simulink model "PilotModelUnitTest"  (R2018b)
settings: Solver=VariableStepAuto  StartTime=0.0  StopTime=100  RelTol=1e-3
values from neighbouring files (symbols this model uses):
  enableHorzMan = 1    [unitTest_PilotModel.m]
  enableVertMan = 0    [unitTest_PilotModel.m]
undefined symbols (not defined in the file or in its folder): ac2dyn_alt0_ft, ac2dyn_con, ac2dyn_lat0_rad, ac2dyn_lon0_rad, daaLogic_turnRate_dps, daaLogic_vertRate_fpm, ddh_ftps2, dh_ftps, dv_ftps2, e_ft, Edot_ftps, h_ft, hdot_ftps, latLonAltState, n_ft, Ndot_ftps, p_radps, phi_rad, phidot_radps, psi_rad, psidot_radps, q_radps, r_radps, theta_rad, thetadot_radps, uasPilot_altitudeK, uasPilot_altitudeOffset, uasPilot_altitudeTheta, uasPilot_coordDelayK, uasPilot_coordDelayMin, uasPilot_coordDelayTheta, uasPilot_desiredTurnRate_dps, uasPilot_desiredVertRate_ftpm, uasPilot_deterministicMode, uasPilot_dt_s, uasPilot_executionDelayMin, uasPilot_executionDelayMu, uasPilot_initialDelayMin, uasPilot_initialDelayMu, uasPilot_maxRelativeHdg, uasPilot_meanUpdateTimes, uasPilot_mentalFilter_climbThresh_fps, uasPilot_mentalFilter_numSamp, uasPilot_mentalFilter_turnThresh_rad, uasPilot_minUpdateTimes, uasPilot_operatorEnabled, uasPilot_probDescend, uasPilot_probFollowMinDev, uasPilot_probLeftTurn, uasPilot_probTurn, uasPilot_reducedClimbAlt_ft, uasPilot_reducedTurnAngle_deg, uasPilot_seedChoose, uasPilot_seedCoordDelay, uasPilot_seedExecutionDelay, uasPilot_seedInitialDelay, uasPilot_seedTurn, uasPilot_seedUpdate, uasPilot_seedVertical, uasPilot_triggerLevel ... (+8)
libraries: simulink x17, NullAircraftEstimateBus x1, uas_pilot_model_r6 x1
(part 2 of 2)

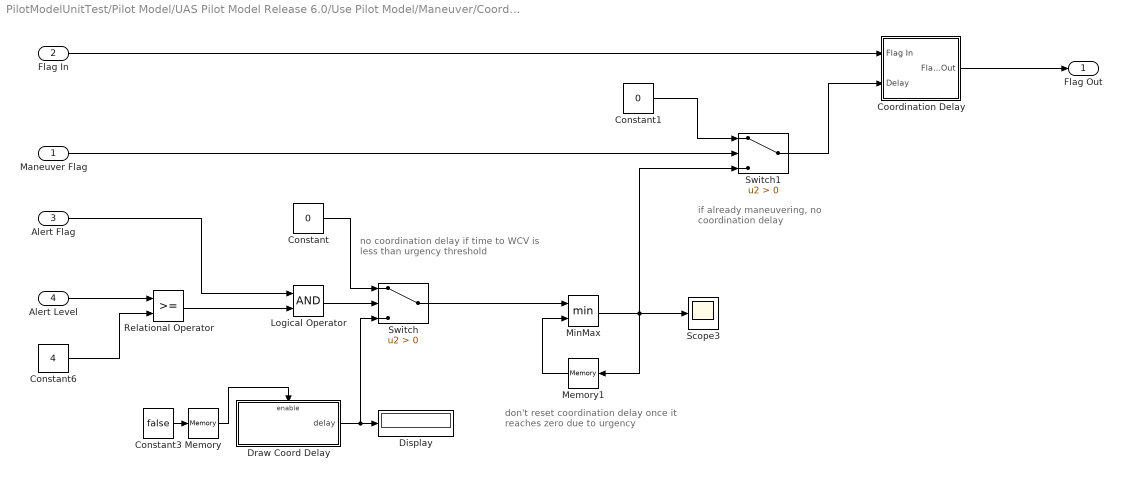
== system PilotModelUnitTest/Pilot Model/UAS Pilot Model Release 6.0/Use Pilot Model/Maneuver/Coordination Delay ==
  note: don't reset coordination delay once
      | it reaches zero due to urgency
  note: no coordination delay if time to WCV
      | is less than urgency threshold
  note: if already maneuvering, no
      | coordination delay
  Maneuver Flag : Inport
  Flag In : Inport  Port=2
  Alert Flag : Inport  Port=3
  Alert Level : Inport  Port=4
  Constant : Constant  Value=0
  Constant1 : Constant  Value=0
  Constant3 : Constant  Value=false
  Constant6 : Constant  Value=4
  Coordination Delay : Subsystem
  Display : Display
  Draw Coord Delay : Subsystem  TreatAsAtomicUnit=on  mask{k=coord_delay_k, theta=coord_delay_theta, offset=coord_delay_min, seed=rng_seed_coord}
      mask prompts: k "Gamma Distribution Shape Parameter, k"; theta "Gamma Distribution Scale Parameter, theta"
  Logical Operator : Logic  AllPortsSameDT=off  OutDataTypeStr=boolean
  Memory : Memory  InitialCondition=true  InheritSampleTime=on
  Memory1 : Memory  InitialCondition=1000  InheritSampleTime=on
  MinMax : MinMax  Inputs=2
  Relational Operator : RelationalOperator  OutDataTypeStr=boolean  RndMeth=Nearest
  Scope3 : Scope
  Switch : Switch  Criteria=u2 > Threshold
  Switch1 : Switch  Criteria=u2 > Threshold
  Flag Out : Outport
  wires:
  Constant3/1 -> Memory/1
  Memory/1 -> Draw Coord Delay/Enable
  Maneuver Flag/1 -> Switch1/2
  Constant1/1 -> Switch1/1
  Switch1/1 -> Coordination Delay/2(Delay)
  Constant/1 -> Switch/1
  Alert Level/1 -> Relational Operator/1
  Coordination Delay/1(Flag Out) -> Flag Out/1
  Relational Operator/1 -> Logical Operator/2
  Constant6/1 -> Relational Operator/2
  Logical Operator/1 -> Switch/2
  Draw Coord Delay/1(delay) -> Switch/3, Display/1
  MinMax/1 -> Memory1/1, Scope3/1, Switch1/3
  Memory1/1 -> MinMax/2
  Switch/1 -> MinMax/1
  Flag In/1 -> Coordination Delay/1(Flag In)
  Alert Flag/1 -> Logical Operator/1

== system PilotModelUnitTest/Pilot Model/UAS Pilot Model Release 6.0/Use Pilot Model/Maneuver/Initial Delay ==
  note: If already maneuvering, no delay
      | for subsequent maneuvers
  Maneuver Flag : Inport
  Alert Flag : Inport  Port=2
  Constant1 : Constant  Value=0
  Constant3 : Constant  Value=false
  Display : Display
  Draw Initial Delay : Subsystem  TreatAsAtomicUnit=on  mask{mu=mean_initial_delay, offset=min_initial_delay, seed=rng_seed_initial}
      mask prompts: mu "Exponential Distribution Mean Parameter, k"
  Memory : Memory  InitialCondition=true  InheritSampleTime=on
  Scope : Scope  NumInputPorts=2
  Switch1 : Switch  Criteria=u2 > Threshold
  Wait for Intruder to Give Way : Subsystem
  Flag Out : Outport
  wires:
  Constant3/1 -> Memory/1
  Memory/1 -> Draw Initial Delay/Enable
  Constant1/1 -> Switch1/1
  Draw Initial Delay/1(delay) -> Display/1, Switch1/3
  Switch1/1 -> Wait for Intruder to Give Way/2(Delay)
  Maneuver Flag/1 -> Switch1/2
  Wait for Intruder to Give Way/1(Flag Out) -> Scope/2, Flag Out/1
  Alert Flag/1 -> Scope/1, Wait for Intruder to Give Way/1(Flag In)

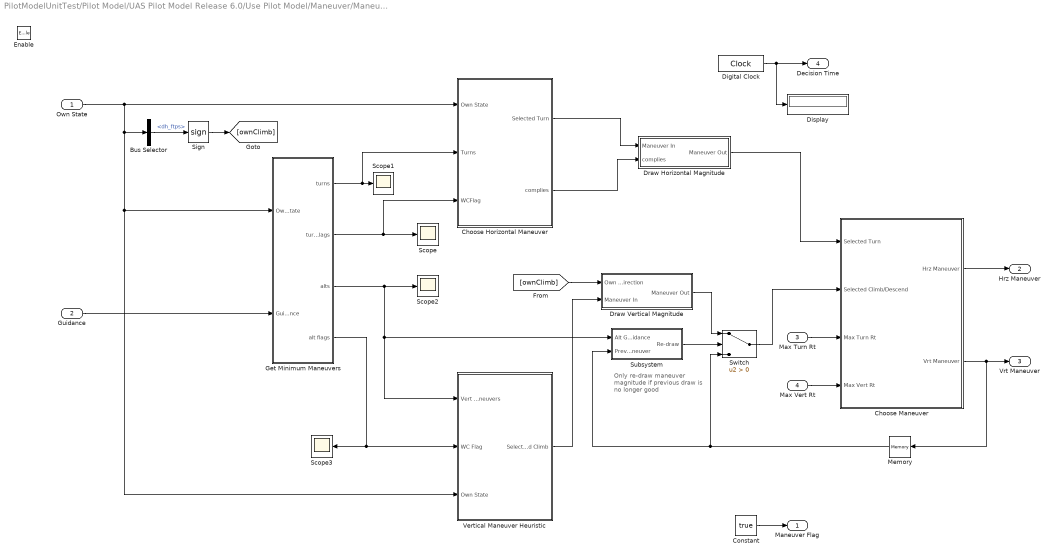
== system PilotModelUnitTest/Pilot Model/UAS Pilot Model Release 6.0/Use Pilot Model/Maneuver/Maneuver Selection ==
  note: Only re-draw maneuver
      | magnitude if previous
      | draw is no longer good
  Own State : Inport
  Guidance : Inport  Port=2
  Max Turn Rt : Inport  Port=3
  Max Vert Rt : Inport  Port=4
  Enable : EnablePort
  Bus Selector : BusSelector  OutputSignals=dh_ftps
  Choose Horizontal Maneuver : Subsystem
  Choose Maneuver : Subsystem
  Constant : Constant  Value=true
  Digital Clock : DigitalClock
  Display : Display
  Draw Horizontal Magnitude : Subsystem
  Draw Vertical Magnitude : Subsystem
  Get Minimum Maneuvers : Subsystem
  Memory : Memory  InheritSampleTime=on
  Scope{,1..3} (4 alike) : Scope
  Sign : Signum
  Subsystem : Subsystem
  Switch : Switch  Criteria=u2 > Threshold
  Vertical Maneuver Heuristic : Subsystem
  Maneuver Flag : Outport  InitialOutput=0
  Hrz Maneuver : Outport  Port=2  OutDataTypeStr=Bus: AvoidanceManeuver  InitialOutput=0
  Vrt Maneuver : Outport  Port=3  OutDataTypeStr=Bus: AvoidanceManeuver  InitialOutput=0
  Decision Time : Outport  Port=4
  wires:
  [ownClimb] -> Draw Vertical Magnitude/1(Own Vertical Direction)
  Sign/1 -> [ownClimb]
  Bus Selector/1 -> Sign/1  "<dh_ftps>"
  Max Vert Rt/1 -> Choose Maneuver/4(Max Vert Rt)
  Max Turn Rt/1 -> Choose Maneuver/3(Max Turn Rt)
  Draw Vertical Magnitude/1(Maneuver Out) -> Switch/1
  Draw Horizontal Magnitude/1(Maneuver Out) -> Choose Maneuver/1(Selected Turn)
  Choose Maneuver/2(Vrt Maneuver) -> Memory/1, Vrt Maneuver/1
  Guidance/1 -> Get Minimum Maneuvers/2(Guidance)
  Vertical Maneuver Heuristic/1(Selected Climb) -> Draw Vertical Magnitude/2(Maneuver In)
  Choose Horizontal Maneuver/1(Selected Turn) -> Draw Horizontal Magnitude/1(Maneuver In)
  Choose Maneuver/1(Hrz Maneuver) -> Hrz Maneuver/1
  Own State/1 -> Bus Selector/1, Vertical Maneuver Heuristic/3(Own State), Get Minimum Maneuvers/1(Own State), Choose Horizontal Maneuver/1(Own State)
  Constant/1 -> Maneuver Flag/1
  Digital Clock/1 -> Decision Time/1, Display/1
  Get Minimum Maneuvers/4(alt flags) -> Scope3/1, Vertical Maneuver Heuristic/2(WC Flag)
  Get Minimum Maneuvers/3(alts) -> Scope2/1, Subsystem/1(Alt Guidance), Vertical Maneuver Heuristic/1(Vert Maneuvers)
  Get Minimum Maneuvers/2(turn flags) -> Scope/1, Choose Horizontal Maneuver/3(WCFlag)
  Get Minimum Maneuvers/1(turns) -> Scope1/1, Choose Horizontal Maneuver/2(Turns)
  Choose Horizontal Maneuver/2(complies) -> Draw Horizontal Magnitude/2(complies)
  Memory/1 -> Switch/3, Subsystem/2(Prev Maneuver)
  Subsystem/1(Re-draw) -> Switch/2
  Switch/1 -> Choose Maneuver/2(Selected Climb/Descend)

== system PilotModelUnitTest/Pilot Model/UAS Pilot Model Release 6.0/Use Pilot Model/Update Delay/Exponential Delay ==
  note: Delay exponentially distributed with mean interarrival time of beta.
      | Delay over (returns true) if X <= 1-exp(-dt/beta) where X is uniformly distributed between 0 and 1.
  beta : Inport
  Constant : Constant
  Divide : Product  Inputs=*/
  Math Function : Math  SaturateOnIntegerOverflow=on
  Relational Operator : RelationalOperator  Operator=<=  OutDataTypeStr=boolean  RndMeth=Nearest
  Sample Time : Constant  Value=dt
  Subtract : Sum  Inputs=+-
  Unary Minus : UnaryMinus
  Uniform Random Number : UniformRandomNumber  Minimum=0  Seed=seed  SampleTime=dt
  Enable : Outport  OutDataTypeStr=boolean
  wires:
  Relational Operator/1 -> Enable/1
  Divide/1 -> Math Function/1
  Uniform Random Number/1 -> Relational Operator/1
  Subtract/1 -> Relational Operator/2
  Math Function/1 -> Subtract/2
  Sample Time/1 -> Unary Minus/1
  Constant/1 -> Subtract/1
  Unary Minus/1 -> Divide/1
  beta/1 -> Divide/2

== system PilotModelUnitTest/Pilot Model/UAS Pilot Model Release 6.0/Use Pilot Model/Update Delay/Fixed Update Delay ==
  Flag In : Inport
  Delay : Inport  Port=2
  Add : Sum
  Constant1 : Constant  Value=0
  Constant2 : Constant
  Memory : Memory  InheritSampleTime=on
  Relational Operator : RelationalOperator  Operator=>  OutDataTypeStr=boolean  RndMeth=Nearest
  Scope1 : Scope
  Scope2 : Scope
  Scope5 : Scope
  Switch : Switch  Criteria=u2 > Threshold
  Flag Out : Outport
  wires:
  Delay/1 -> Scope2/1, Relational Operator/2
  Relational Operator/1 -> Scope1/1, Flag Out/1
  Switch/1 -> Memory/1, Relational Operator/1
  Constant1/1 -> Switch/3
  Memory/1 -> Add/2
  Flag In/1 -> Switch/2
  Constant2/1 -> Add/1
  Add/1 -> Scope5/1, Switch/1

== system PilotModelUnitTest/Pilot Model/UAS Pilot Model Release 6.0/Use Pilot Model/Update Delay/Mean Time to Update ==
  Constant : Constant  Value=20
  Constant1 : Constant  Value=3
  Constant2 : Constant  Value=20
  Constant3 : Constant  Value=20
  Constant4 : Constant  Value=5
  Constant5 : Constant  Value=3
  Mux : Mux  Inputs=6
  Mean Time : Outport
  wires:
  Constant1/1 -> Mux/6
  Constant2/1 -> Mux/2
  Constant4/1 -> Mux/4
  Constant5/1 -> Mux/5
  Constant3/1 -> Mux/3
  Constant/1 -> Mux/1
  Mux/1 -> Mean Time/1

== system PilotModelUnitTest/Pilot Model/UAS Pilot Model Release 6.0/Use Pilot Model/Update Delay/Minimum Time to Update ==
  Constant : Constant  Value=15
  Constant1 : Constant  Value=5
  Constant2 : Constant  Value=15
  Constant3 : Constant  Value=15
  Constant4 : Constant  Value=5
  Constant5 : Constant  Value=5
  Mux : Mux  Inputs=6
  Min Time : Outport
  wires:
  Constant1/1 -> Mux/6
  Constant2/1 -> Mux/2
  Constant4/1 -> Mux/4
  Constant5/1 -> Mux/5
  Constant3/1 -> Mux/3
  Constant/1 -> Mux/1
  Mux/1 -> Min Time/1

== system PilotModelUnitTest/Pilot Model/UAS Pilot Model Release 6.0/Use Pilot Model/Execution Delay/Subsystem/Exponential Delay ==
  note: Delay exponentially distributed with mean interarrival time of beta.
      | Delay over (returns true) if X <= 1-exp(-dt/beta) where X is uniformly distributed between 0 and 1.
  beta : Inport
  Constant : Constant
  Divide : Product  Inputs=*/
  Math Function : Math  SaturateOnIntegerOverflow=on
  Relational Operator : RelationalOperator  Operator=<=  OutDataTypeStr=boolean  RndMeth=Nearest
  Sample Time : Constant  Value=dt
  Subtract : Sum  Inputs=+-
  Unary Minus : UnaryMinus
  Uniform Random Number : UniformRandomNumber  Minimum=0  Seed=seed  SampleTime=dt
  Enable : Outport  OutDataTypeStr=boolean
  wires:
  Relational Operator/1 -> Enable/1
  Divide/1 -> Math Function/1
  Uniform Random Number/1 -> Relational Operator/1
  Subtract/1 -> Relational Operator/2
  Math Function/1 -> Subtract/2
  Sample Time/1 -> Unary Minus/1
  Constant/1 -> Subtract/1
  Unary Minus/1 -> Divide/1
  beta/1 -> Divide/2

== system PilotModelUnitTest/Pilot Model/UAS Pilot Model Release 6.0/Use Pilot Model/Execution Delay/Subsystem/Fixed Update Delay ==
  Flag In : Inport
  Delay : Inport  Port=2
  Add : Sum
  Constant1 : Constant  Value=0
  Constant2 : Constant
  Memory : Memory  InheritSampleTime=on
  Relational Operator : RelationalOperator  Operator=>  OutDataTypeStr=boolean  RndMeth=Nearest
  Switch : Switch  Criteria=u2 > Threshold
  Flag Out : Outport
  wires:
  Delay/1 -> Relational Operator/2
  Relational Operator/1 -> Flag Out/1
  Switch/1 -> Memory/1, Relational Operator/1
  Constant1/1 -> Switch/3
  Memory/1 -> Add/2
  Flag In/1 -> Switch/2
  Constant2/1 -> Add/1
  Add/1 -> Switch/1

== system PilotModelUnitTest/Pilot Model/UAS Pilot Model Release 6.0/Use Pilot Model/Maneuver/Coordination Delay/Coordination Delay ==
  Flag In : Inport
  Delay : Inport  Port=2
  Add : Sum
  Constant1 : Constant  Value=0
  Constant2 : Constant
  Memory : Memory  InheritSampleTime=on
  Relational Operator : RelationalOperator  Operator=>  OutDataTypeStr=boolean  RndMeth=Nearest
  Switch : Switch  Criteria=u2 > Threshold
  Flag Out : Outport
  wires:
  Delay/1 -> Relational Operator/2
  Relational Operator/1 -> Flag Out/1
  Switch/1 -> Memory/1, Relational Operator/1
  Constant1/1 -> Switch/3
  Memory/1 -> Add/2
  Flag In/1 -> Switch/2
  Constant2/1 -> Add/1
  Add/1 -> Switch/1

== system PilotModelUnitTest/Pilot Model/UAS Pilot Model Release 6.0/Use Pilot Model/Maneuver/Coordination Delay/Draw Coord Delay ==
  Enable : EnablePort
  Generate Random Gamma Deviate : Subsystem  mask{k=k, theta=theta, offset=offset, seed=seed}
      mask prompts: k "Shape Parameter, k"; theta "Scale Parameter, theta"
  Rounding Function : Rounding  Operator=round
  delay : Outport  InitialOutput=0
  wires:
  Rounding Function/1 -> delay/1
  Generate Random Gamma Deviate/1(y) -> Rounding Function/1

== system PilotModelUnitTest/Pilot Model/UAS Pilot Model Release 6.0/Use Pilot Model/Maneuver/Initial Delay/Draw Initial Delay ==
  Enable : EnablePort
  Generate Random Exponential Deviate : Subsystem  mask{mu=mu, offset=offset, seed=seed}
      mask prompts: mu "Mean Parameter, mu"
  Rounding Function : Rounding  Operator=round
  delay : Outport  InitialOutput=0
  wires:
  Generate Random Exponential Deviate/1(y) -> Rounding Function/1
  Rounding Function/1 -> delay/1

== system PilotModelUnitTest/Pilot Model/UAS Pilot Model Release 6.0/Use Pilot Model/Maneuver/Initial Delay/Wait for Intruder to Give Way ==
  Flag In : Inport
  Delay : Inport  Port=2
  Add : Sum
  Constant1 : Constant  Value=0
  Constant2 : Constant
  Memory : Memory  InheritSampleTime=on
  Relational Operator : RelationalOperator  Operator=>  OutDataTypeStr=boolean  RndMeth=Nearest
  Scope : Scope
  Switch : Switch  Criteria=u2 > Threshold
  Flag Out : Outport
  wires:
  Delay/1 -> Relational Operator/2
  Relational Operator/1 -> Flag Out/1
  Switch/1 -> Memory/1, Relational Operator/1
  Constant1/1 -> Switch/3
  Memory/1 -> Add/2
  Flag In/1 -> Switch/2
  Constant2/1 -> Add/1
  Add/1 -> Scope/1, Switch/1

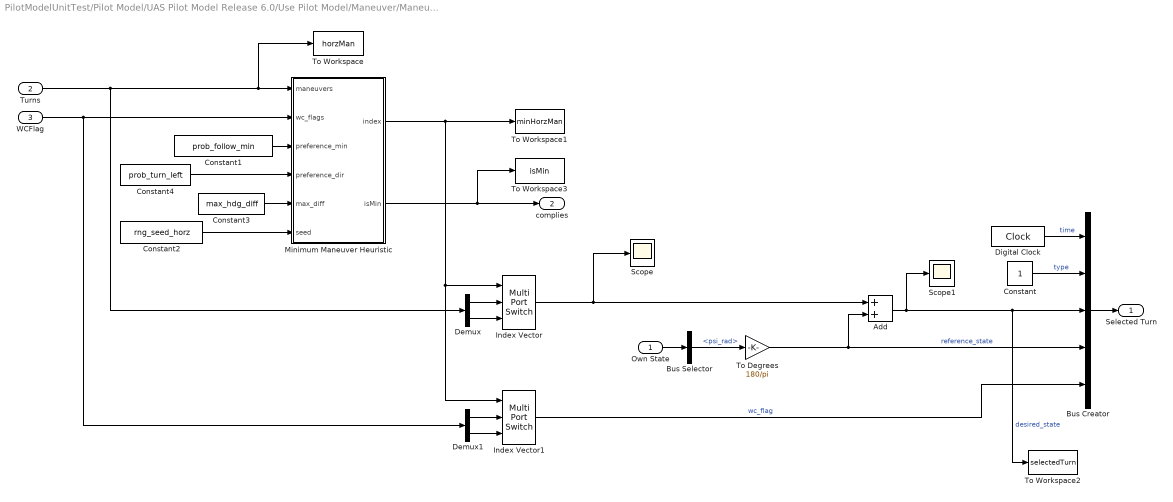
== system PilotModelUnitTest/Pilot Model/UAS Pilot Model Release 6.0/Use Pilot Model/Maneuver/Maneuver Selection/Choose Horizontal Maneuver ==
  Own State : Inport
  Turns : Inport  Port=2
  WCFlag : Inport  Port=3
  Add : Sum
  Bus Selector : BusSelector  OutputSignals=psi_rad
  Bus Creator : BusCreator  Inputs=5  OutDataTypeStr=Bus: AvoidanceManeuver
  Constant : Constant
  Constant1 : Constant  Value=prob_follow_min
  Constant2 : Constant  Value=rng_seed_horz
  Constant3 : Constant  Value=max_hdg_diff
  Constant4 : Constant  Value=prob_turn_left
  Demux : Demux  Outputs=2
  Demux1 : Demux  Outputs=2
  Digital Clock : DigitalClock  SampleTime=dt
  Index Vector : MultiPortSwitch  DataPortOrder=Specify indices  Inputs=2  DataPortIndices={1,2}
  Index Vector1 : MultiPortSwitch  DataPortOrder=Specify indices  Inputs=2  DataPortIndices={1,2}
  Minimum Maneuver Heuristic : MATLAB Function  TreatAsAtomicUnit=on
  Scope : Scope
  Scope1 : Scope
  To Degrees : Gain  Gain=180/pi
  To Workspace : ToWorkspace  VariableName=horzMan  SaveFormat=Timeseries  SampleTime=-1
  To Workspace1 : ToWorkspace  VariableName=minHorzMan  SaveFormat=Timeseries  SampleTime=-1
  To Workspace2 : ToWorkspace  VariableName=selectedTurn  SaveFormat=Timeseries  SampleTime=-1
  To Workspace3 : ToWorkspace  VariableName=isMin  SaveFormat=Timeseries  SampleTime=-1
  Selected Turn : Outport  OutDataTypeStr=Bus: AvoidanceManeuver
  complies : Outport  Port=2
  wires:
  Add/1 -> Scope1/1, To Workspace2/1, Bus Creator/3  "desired_state"
  To Degrees/1 -> Add/2, Bus Creator/4  "reference_state"
  Constant4/1 -> Minimum Maneuver Heuristic/4(preference_dir)
  Constant3/1 -> Minimum Maneuver Heuristic/5(max_diff)
  Demux1/2 -> Index Vector1/3
  Demux1/1 -> Index Vector1/2
  Demux/2 -> Index Vector/3
  Demux/1 -> Index Vector/2
  Minimum Maneuver Heuristic/1(index) -> Index Vector/1, Index Vector1/1, To Workspace1/1
  Constant2/1 -> Minimum Maneuver Heuristic/6(seed)
  Constant1/1 -> Minimum Maneuver Heuristic/3(preference_min)
  Bus Selector/1 -> To Degrees/1  "<psi_rad>"
  Own State/1 -> Bus Selector/1
  Constant/1 -> Bus Creator/2  "type"
  Index Vector/1 -> Add/1, Scope/1
  Index Vector1/1 -> Bus Creator/5  "wc_flag"
  Digital Clock/1 -> Bus Creator/1  "time"
  Bus Creator/1 -> Selected Turn/1
  Turns/1 -> To Workspace/1, Minimum Maneuver Heuristic/1(maneuvers), Demux/1
  WCFlag/1 -> Minimum Maneuver Heuristic/2(wc_flags), Demux1/1
  Minimum Maneuver Heuristic/2(isMin) -> To Workspace3/1, complies/1

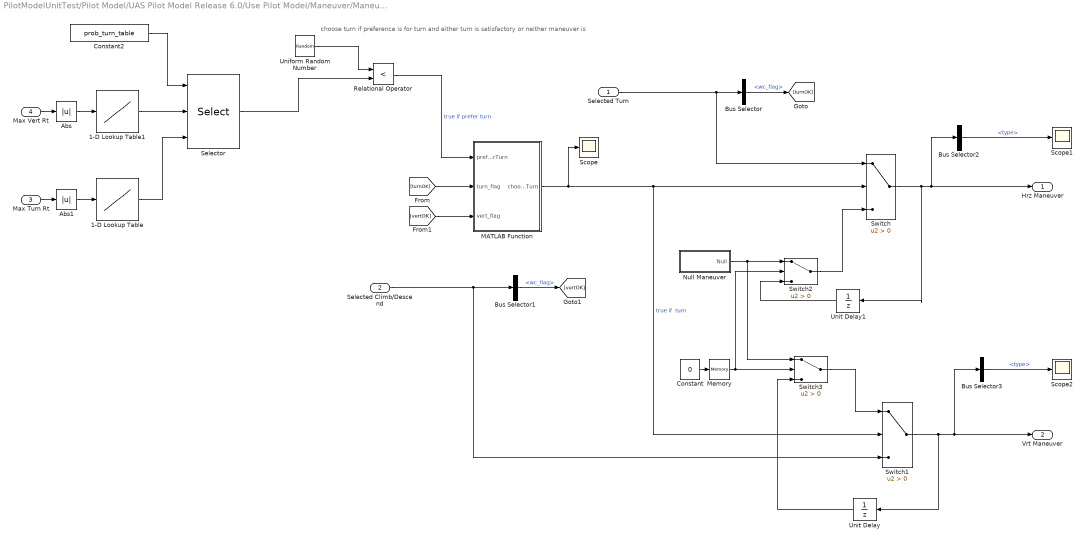
== system PilotModelUnitTest/Pilot Model/UAS Pilot Model Release 6.0/Use Pilot Model/Maneuver/Maneuver Selection/Choose Maneuver ==
  note: choose turn if preference is for turn and either turn is satisfactory or neither maneuver is
  Selected Turn : Inport
  Selected Climb/Descend : Inport  Port=2
  Max Turn Rt : Inport  Port=3
  Max Vert Rt : Inport  Port=4
  1-D Lookup Table : Lookup_n-D  NumberOfTableDimensions=1  BreakpointsForDimension1=[-1,0+1e-6,2+1e-6]  Table=[1,2,3]  InterpMethod=Flat  InternalRulePriority=Speed  RndMeth=Simplest  InputSameDT=on
  1-D Lookup Table1 : Lookup_n-D  NumberOfTableDimensions=1  BreakpointsForDimension1=[-1,0+1e-6,1000+1e-6]  Table=[1,2,3]  InterpMethod=Flat  InternalRulePriority=Speed  RndMeth=Simplest  InputSameDT=on
  Abs : Abs
  Abs1 : Abs
  Bus Selector2 : BusSelector  OutputSignals=type
  Bus Selector3 : BusSelector  OutputSignals=type
  Bus Selector : BusSelector  OutputSignals=wc_flag
  Bus Selector1 : BusSelector  OutputSignals=wc_flag
  Constant : Constant  Value=0
  Constant2 : Constant  Value=prob_turn_table
  MATLAB Function : MATLAB Function  TreatAsAtomicUnit=on
  Memory : Memory  InitialCondition=1  InheritSampleTime=on
  Null Maneuver : Subsystem
  Relational Operator : RelationalOperator  Operator=<  OutDataTypeStr=boolean  RndMeth=Nearest
  Scope : Scope
  Scope1 : Scope
  Scope2 : Scope
  Selector : Selector  NumberOfDimensions=2  InputPortWidth=3  IndexOptions=Index vector (port),Index vector (port)  Indices=[1 3],1  OutputSizes=1,1
  Switch{,1..3} (4 alike) : Switch  Criteria=u2 > Threshold
  Uniform Random Number : UniformRandomNumber  Minimum=0  Seed=rng_seed_horz_vs_vert  SampleTime=1
  Unit Delay : UnitDelay  SampleTime=-1
  Unit Delay1 : UnitDelay  SampleTime=-1
  Hrz Maneuver : Outport
  Vrt Maneuver : Outport  Port=2
  wires:
  Max Vert Rt/1 -> Abs/1
  Max Turn Rt/1 -> Abs1/1
  1-D Lookup Table/1 -> Selector/3
  1-D Lookup Table1/1 -> Selector/2
  Abs1/1 -> 1-D Lookup Table/1
  Abs/1 -> 1-D Lookup Table1/1
  Constant2/1 -> Selector/1
  Bus Selector3/1 -> Scope2/1  "<type>"
  Switch1/1 -> Vrt Maneuver/1, Bus Selector3/1, Unit Delay/1
  Bus Selector2/1 -> Scope1/1  "<type>"
  Unit Delay1/1 -> Switch2/3
  Unit Delay/1 -> Switch3/3
  Switch3/1 -> Switch1/1
  Null Maneuver/1(Null) -> Switch3/1, Switch2/1
  Switch2/1 -> Switch/3
  Memory/1 -> Switch3/2, Switch2/2
  Constant/1 -> Memory/1
  Switch/1 -> Hrz Maneuver/1, Bus Selector2/1, Unit Delay1/1
  [turnOK] -> MATLAB Function/2(turn_flag)
  [vertOK] -> MATLAB Function/3(vert_flag)
  MATLAB Function/1(chooseTurn) -> Switch/2, Switch1/2, Scope/1  "true if  turn"
  Relational Operator/1 -> MATLAB Function/1(preferTurn)  "true if prefer turn"
  Bus Selector1/1 -> [vertOK]  "<wc_flag>"
  Bus Selector/1 -> [turnOK]  "<wc_flag>"
  Uniform Random Number/1 -> Relational Operator/1
  Selected Turn/1 -> Bus Selector/1, Switch/1
  Selected Climb/Descend/1 -> Bus Selector1/1, Switch1/3
  Selector/1 -> Relational Operator/2

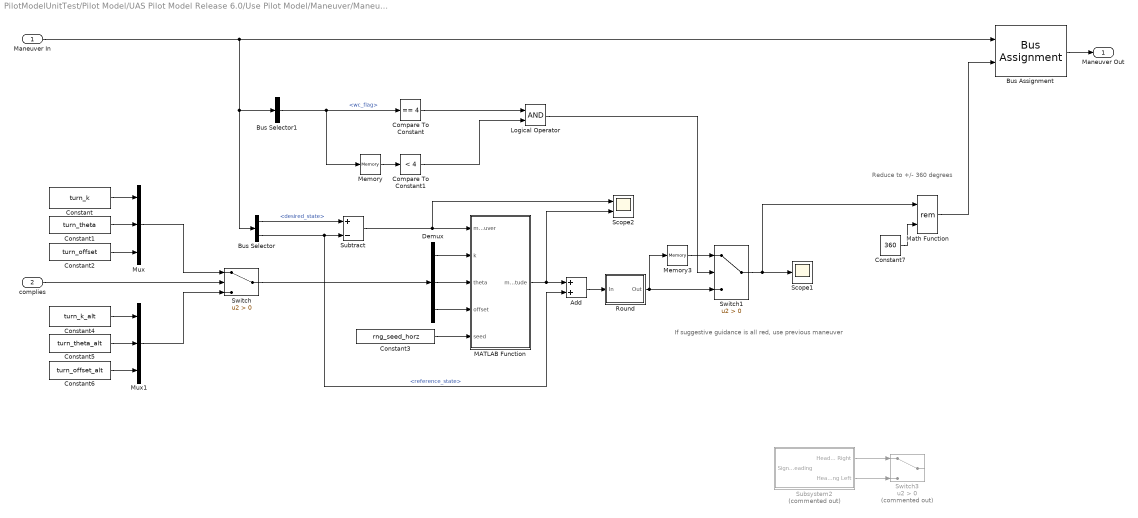
== system PilotModelUnitTest/Pilot Model/UAS Pilot Model Release 6.0/Use Pilot Model/Maneuver/Maneuver Selection/Draw Horizontal Magnitude ==
  note: If suggestive guidance is all red, use previous maneuver
  note: Reduce to +/- 360 degrees
  Maneuver In : Inport
  complies : Inport  Port=2
  Add : Sum
  Bus Assignment : BusAssignment  AssignedSignals=desired_state
  Bus Selector : BusSelector  OutputSignals=desired_state,reference_state
  Bus Selector1 : BusSelector  OutputSignals=wc_flag
  Compare To Constant : simulink/Logic and Bit Operations/Compare To Constant  relop===  const=4  OutDataTypeStr=boolean
  Compare To Constant1 : simulink/Logic and Bit Operations/Compare To Constant  relop=<  const=4  OutDataTypeStr=boolean
  Constant : Constant  Value=turn_k
  Constant1 : Constant  Value=turn_theta
  Constant2 : Constant  Value=turn_offset
  Constant3 : Constant  Value=rng_seed_horz
  Constant4 : Constant  Value=turn_k_alt
  Constant5 : Constant  Value=turn_theta_alt
  Constant6 : Constant  Value=turn_offset_alt
  Constant7 : Constant  Value=360
  Demux : Demux  Outputs=3
  Logical Operator : Logic  AllPortsSameDT=off  OutDataTypeStr=boolean
  MATLAB Function : MATLAB Function  TreatAsAtomicUnit=on
  Math Function : Math  Operator=rem  SaturateOnIntegerOverflow=on
  Memory : Memory  InitialCondition=4  InheritSampleTime=on
  Memory3 : Memory  InheritSampleTime=on
  Mux : Mux  Inputs=3
  Mux1 : Mux  Inputs=3
  Round : Subsystem  mask{factor=5}
      mask prompts: factor "Round to nearest:"
  Scope1 : Scope
  Scope2 : Scope  NumInputPorts=2
  Subsystem2 : Subsystem  Commented=on
  Subtract : Sum  Inputs=+-
  Switch : Switch  Criteria=u2 > Threshold
  Switch1 : Switch  Criteria=u2 > Threshold
  Switch3 : Switch  Commented=on  Criteria=u2 > Threshold
  Maneuver Out : Outport
  wires:
  Constant7/1 -> Math Function/2
  Subsystem2/2(Heading Left) -> Switch3/3
  Subsystem2/1(Heading Right) -> Switch3/1
  Math Function/1 -> Bus Assignment/2
  Bus Assignment/1 -> Maneuver Out/1
  Add/1 -> Round/1(In)
  MATLAB Function/1(magnitude) -> Scope2/2, Add/1
  Constant3/1 -> MATLAB Function/5(seed)
  Demux/3 -> MATLAB Function/4(offset)
  Demux/2 -> MATLAB Function/3(theta)
  Demux/1 -> MATLAB Function/2(k)
  Subtract/1 -> Scope2/1, MATLAB Function/1(maneuver)
  Bus Selector/2 -> Subtract/2, Add/2  "<reference_state>"
  Bus Selector/1 -> Subtract/1  "<desired_state>"
  Round/1(Out) -> Memory3/1, Switch1/3
  Constant/1 -> Mux/1
  Constant1/1 -> Mux/2
  Constant2/1 -> Mux/3
  Constant4/1 -> Mux1/1
  Constant5/1 -> Mux1/2
  Constant6/1 -> Mux1/3
  Mux1/1 -> Switch/3
  Mux/1 -> Switch/1
  complies/1 -> Switch/2
  Switch/1 -> Demux/1
  Bus Selector1/1 -> Memory/1, Compare To Constant/1  "<wc_flag>"
  Switch1/1 -> Scope1/1, Math Function/1
  Memory/1 -> Compare To Constant1/1
  Compare To Constant1/1 -> Logical Operator/2
  Logical Operator/1 -> Switch1/2
  Maneuver In/1 -> Bus Selector/1, Bus Selector1/1, Bus Assignment/1
  Compare To Constant/1 -> Logical Operator/1
  Memory3/1 -> Switch1/1

== system PilotModelUnitTest/Pilot Model/UAS Pilot Model Release 6.0/Use Pilot Model/Maneuver/Maneuver Selection/Draw Vertical Magnitude ==
  Own Vertical Direction : Inport
  Maneuver In : Inport  Port=2
  Altitude Floor : Subsystem  mask{alt_floor=500}
      mask prompts: alt_floor "Altitude Floor (feet)"
  Bus Assignment : BusAssignment  AssignedSignals=desired_state
  Bus Selector : BusSelector  OutputSignals=desired_state,reference_state
  Constant : Constant  Value=alt_k
  Constant1 : Constant  Value=alt_theta
  Constant2 : Constant  Value=alt_offset
  Constant3 : Constant  Value=rng_seed_vert
  MATLAB Function : MATLAB Function  TreatAsAtomicUnit=on
  Round Altitude : Subsystem
  Subtract : Sum  Inputs=+-
  Maneuver Out : Outport
  wires:
  Own Vertical Direction/1 -> Round Altitude/3(Ownship Climb/Descend)
  Round Altitude/1(Alt Out) -> Altitude Floor/1(Alt In)
  MATLAB Function/1(magnitude) -> Round Altitude/1(Alt In)
  Altitude Floor/1(Alt Out) -> Bus Assignment/2
  Constant3/1 -> MATLAB Function/5(seed)
  Constant2/1 -> MATLAB Function/4(offset)
  Constant1/1 -> MATLAB Function/3(theta)
  Constant/1 -> MATLAB Function/2(k)
  Subtract/1 -> MATLAB Function/1(maneuver)  "minimum maneuver"
  Bus Selector/2 -> Subtract/2, Round Altitude/2(Reference Alt), Altitude Floor/2(Reference Alt)  "<reference_state>"
  Bus Selector/1 -> Subtract/1  "<desired_state>"
  Maneuver In/1 -> Bus Selector/1, Bus Assignment/1
  Bus Assignment/1 -> Maneuver Out/1

== system PilotModelUnitTest/Pilot Model/UAS Pilot Model Release 6.0/Use Pilot Model/Maneuver/Maneuver Selection/Get Minimum Maneuvers ==
  Own State : Inport
  Guidance : Inport  Port=2
  Bus Selector : BusSelector  OutputSignals=h_ft
  Get Minimum Altitudes : MATLAB Function  TreatAsAtomicUnit=on
  Get Minimum Turns : MATLAB Function  TreatAsAtomicUnit=on
  Scope : Scope
  To Workspace : ToWorkspace  VariableName=minTurn  SaveFormat=Timeseries  SampleTime=-1
  To Workspace1 : ToWorkspace  VariableName=minAlt  SaveFormat=Timeseries  SampleTime=-1
  To Workspace2 : ToWorkspace  VariableName=turnFlags  SaveFormat=Timeseries  SampleTime=-1
  To Workspace3 : ToWorkspace  VariableName=altFlags  SaveFormat=Timeseries  SampleTime=-1
  turns : Outport
  turn flags : Outport  Port=2
  alts : Outport  Port=3
  alt flags : Outport  Port=4
  wires:
  Get Minimum Altitudes/2(wc_flag) -> To Workspace3/1, alt flags/1
  Get Minimum Altitudes/1(alts) -> To Workspace1/1, alts/1
  Get Minimum Turns/2(wc_flag) -> To Workspace2/1, turn flags/1
  Get Minimum Turns/1(turns) -> To Workspace/1, turns/1
  Guidance/1 -> Scope/1, Get Minimum Turns/1(bands), Get Minimum Altitudes/1(bands)
  Own State/1 -> Bus Selector/1
  Bus Selector/1 -> Get Minimum Altitudes/2(currAlt)  "<h_ft>"

== system PilotModelUnitTest/Pilot Model/UAS Pilot Model Release 6.0/Use Pilot Model/Maneuver/Maneuver Selection/Subsystem ==
  Alt Guidance : Inport
  Prev Maneuver : Inport  Port=2
  Bus Selector : BusSelector  OutputSignals=desired_state
  Bus Selector1 : BusSelector  OutputSignals=type
  Compare To Zero : simulink/Logic and Bit Operations/Compare To Zero  relop=>  OutDataTypeStr=boolean
  Demux : Demux  Outputs=2
  Logical Operator : Logic  Operator=OR  AllPortsSameDT=off  OutDataTypeStr=boolean
  Logical Operator1 : Logic  AllPortsSameDT=off  OutDataTypeStr=boolean
  Logical Operator2 : Logic  Operator=NOT  AllPortsSameDT=off  OutDataTypeStr=boolean
  Relational Operator : RelationalOperator  OutDataTypeStr=boolean  RndMeth=Nearest
  Relational Operator1 : RelationalOperator  OutDataTypeStr=boolean  RndMeth=Nearest
  Scope{,1..3} (4 alike) : Scope
  Re-draw : Outport
  wires:
  Prev Maneuver/1 -> Bus Selector1/1, Bus Selector/1
  Alt Guidance/1 -> Demux/1
  Demux/1 -> Scope2/1, Relational Operator1/1  "descend"
  Bus Selector/1 -> Scope1/1, Relational Operator/1, Relational Operator1/2  "<desired_state>"
  Demux/2 -> Scope3/1, Relational Operator/2  "climb"
  Relational Operator1/1 -> Logical Operator/1
  Relational Operator/1 -> Logical Operator/2
  Bus Selector1/1 -> Compare To Zero/1  "<type>"
  Compare To Zero/1 -> Logical Operator1/1
  Logical Operator/1 -> Logical Operator1/2
  Logical Operator1/1 -> Logical Operator2/1
  Logical Operator2/1 -> Scope/1, Re-draw/1

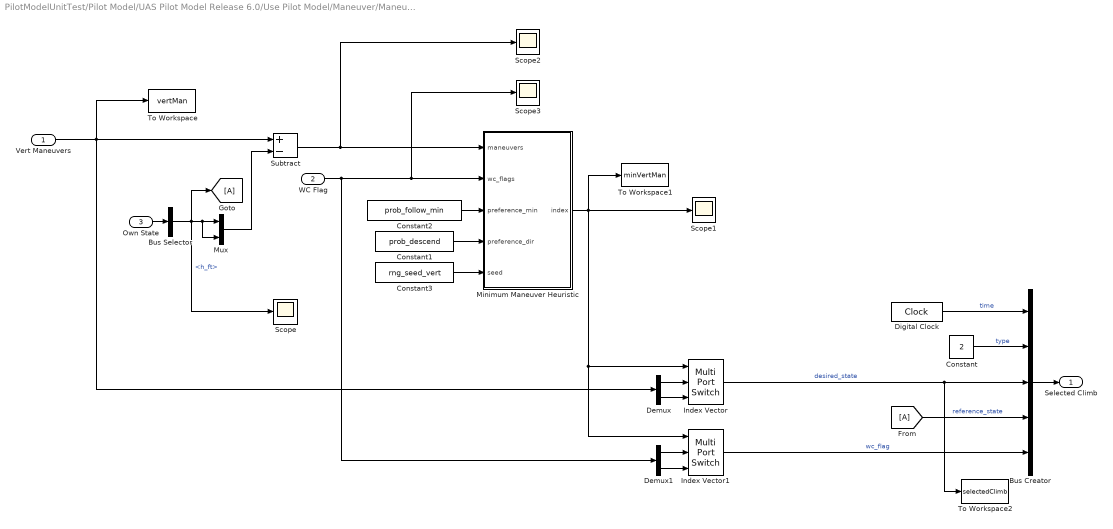
== system PilotModelUnitTest/Pilot Model/UAS Pilot Model Release 6.0/Use Pilot Model/Maneuver/Maneuver Selection/Vertical Maneuver Heuristic ==
  Vert Maneuvers : Inport
  WC Flag : Inport  Port=2
  Own State : Inport  Port=3
  Bus Selector : BusSelector  OutputSignals=h_ft
  Bus Creator : BusCreator  Inputs=5  OutDataTypeStr=Bus: AvoidanceManeuver
  Constant : Constant  Value=2
  Constant1 : Constant  Value=prob_descend
  Constant2 : Constant  Value=prob_follow_min
  Constant3 : Constant  Value=rng_seed_vert
  Demux : Demux  Outputs=2
  Demux1 : Demux  Outputs=2
  Digital Clock : DigitalClock  SampleTime=dt
  Index Vector : MultiPortSwitch  DataPortOrder=Specify indices  Inputs=1  DataPortIndices={1,2}
  Index Vector1 : MultiPortSwitch  DataPortOrder=Specify indices  Inputs=1  DataPortIndices={1,2}
  Minimum Maneuver Heuristic : MATLAB Function  TreatAsAtomicUnit=on
  Mux : Mux  Inputs=2
  Scope{,1..3} (4 alike) : Scope
  Subtract : Sum  Inputs=+-
  To Workspace : ToWorkspace  VariableName=vertMan  SaveFormat=Timeseries  SampleTime=-1
  To Workspace1 : ToWorkspace  VariableName=minVertMan  SaveFormat=Timeseries  SampleTime=-1
  To Workspace2 : ToWorkspace  VariableName=selectedClimb  SaveFormat=Timeseries  SampleTime=-1
  Selected Climb : Outport
  wires:
  Constant1/1 -> Minimum Maneuver Heuristic/4(preference_dir)
  Demux1/2 -> Index Vector1/3
  Demux1/1 -> Index Vector1/2
  Demux/1 -> Index Vector/2
  Demux/2 -> Index Vector/3
  Index Vector1/1 -> Bus Creator/5  "wc_flag"
  Minimum Maneuver Heuristic/1(index) -> To Workspace1/1, Scope1/1, Index Vector1/1, Index Vector/1
  WC Flag/1 -> Scope3/1, Minimum Maneuver Heuristic/2(wc_flags), Demux1/1
  Subtract/1 -> Scope2/1, Minimum Maneuver Heuristic/1(maneuvers)
  Mux/1 -> Subtract/2
  Constant3/1 -> Minimum Maneuver Heuristic/5(seed)
  Constant2/1 -> Minimum Maneuver Heuristic/3(preference_min)
  [A] -> Bus Creator/4  "reference_state"
  Bus Selector/1 -> Scope/1, Mux/1, Mux/2, [A]  "<h_ft>"
  Own State/1 -> Bus Selector/1
  Constant/1 -> Bus Creator/2  "type"
  Digital Clock/1 -> Bus Creator/1  "time"
  Bus Creator/1 -> Selected Climb/1
  Index Vector/1 -> To Workspace2/1, Bus Creator/3  "desired_state"
  Vert Maneuvers/1 -> To Workspace/1, Subtract/1, Demux/1

== system PilotModelUnitTest/Pilot Model/UAS Pilot Model Release 6.0/Use Pilot Model/Maneuver/Coordination Delay/Draw Coord Delay/Generate Random Gamma Deviate ==
  Add : Sum
  Constant : Constant  Value=offset
  MATLAB Function : MATLAB Function  TreatAsAtomicUnit=on
  Scale Parameter : Constant  Value=theta
  Seed : Constant  Value=seed
  Shape Parameter : Constant  Value=k
  y : Outport
  wires:
  Constant/1 -> Add/2
  Add/1 -> y/1
  Seed/1 -> MATLAB Function/3(seed)
  Scale Parameter/1 -> MATLAB Function/2(b)
  MATLAB Function/1(y) -> Add/1
  Shape Parameter/1 -> MATLAB Function/1(a)

== system PilotModelUnitTest/Pilot Model/UAS Pilot Model Release 6.0/Use Pilot Model/Maneuver/Initial Delay/Draw Initial Delay/Generate Random Exponential Deviate ==
  Add : Sum
  Constant : Constant  Value=offset
  MATLAB Function : MATLAB Function  TreatAsAtomicUnit=on
  Mean Parameter : Constant  Value=mu
  Seed : Constant  Value=seed
  y : Outport
  wires:
  Add/1 -> y/1
  Constant/1 -> Add/2
  Seed/1 -> MATLAB Function/2(seed)
  MATLAB Function/1(y) -> Add/1
  Mean Parameter/1 -> MATLAB Function/1(a)

== system PilotModelUnitTest/Pilot Model/UAS Pilot Model Release 6.0/Use Pilot Model/Maneuver/Maneuver Selection/Choose Maneuver/Null Maneuver ==
  Bus Creator : BusCreator  Inputs=5  OutDataTypeStr=Bus: AvoidanceManeuver
  Constant{,1..3} (4 alike) : Constant  Value=0
  Digital Clock : DigitalClock  SampleTime=dt
  Null : Outport
  wires:
  Constant3/1 -> Bus Creator/4  "reference_state"
  Bus Creator/1 -> Null/1
  Digital Clock/1 -> Bus Creator/1  "time"
  Constant1/1 -> Bus Creator/3  "desired_state"
  Constant/1 -> Bus Creator/2  "type"
  Constant2/1 -> Bus Creator/5  "wc_flag"

== system PilotModelUnitTest/Pilot Model/UAS Pilot Model Release 6.0/Use Pilot Model/Maneuver/Maneuver Selection/Draw Horizontal Magnitude/Round ==
  In : Inport
  Constant : Constant  Value=factor
  Divide : Product  Inputs=*/
  Product : Product
  Rounding Function : Rounding  Operator=round
  Out : Outport
  wires:
  Rounding Function/1 -> Product/1
  In/1 -> Divide/1
  Divide/1 -> Rounding Function/1
  Constant/1 -> Product/2, Divide/2
  Product/1 -> Out/1

== system PilotModelUnitTest/Pilot Model/UAS Pilot Model Release 6.0/Use Pilot Model/Maneuver/Maneuver Selection/Draw Horizontal Magnitude/Subsystem2 ==
  Signed Heading : Inport
  Add : Sum
  Add1 : Sum  Inputs=+-
  Constant : Constant  Value=360
  Constant1 : Constant  Value=360
  Constant5 : Constant  Value=360
  Math Function : Math  Operator=rem  SaturateOnIntegerOverflow=on
  Switch : Switch  Criteria=u2 > Threshold
  Heading Right : Outport
  Heading Left : Outport  Port=2
  wires:
  Add1/1 -> Heading Left/1
  Constant1/1 -> Add1/2
  Switch/1 -> Heading Right/1, Add1/1
  Constant/1 -> Add/2
  Math Function/1 -> Switch/2, Switch/1, Add/1
  Signed Heading/1 -> Math Function/1
  Constant5/1 -> Math Function/2
  Add/1 -> Switch/3

== system PilotModelUnitTest/Pilot Model/UAS Pilot Model Release 6.0/Use Pilot Model/Maneuver/Maneuver Selection/Draw Vertical Magnitude/Altitude Floor ==
  note: If the reference altitude is > 500 ft, don't let the commanded
      | altitude be anything less than 500 ft.
  Alt In : Inport
  Reference Alt : Inport  Port=2
  Constant4 : Constant  Value=alt_floor
  MinMax : MinMax  Function=max  Inputs=2
  Relational Operator : RelationalOperator  Operator=<=  OutDataTypeStr=boolean  RndMeth=Nearest
  Switch : Switch  Criteria=u2 > Threshold
  Alt Out : Outport
  wires:
  Reference Alt/1 -> Relational Operator/1
  Switch/1 -> Alt Out/1
  MinMax/1 -> Switch/3
  Alt In/1 -> Switch/1, MinMax/1
  Constant4/1 -> MinMax/2, Relational Operator/2
  Relational Operator/1 -> Switch/2

== system PilotModelUnitTest/Pilot Model/UAS Pilot Model Release 6.0/Use Pilot Model/Maneuver/Maneuver Selection/Draw Vertical Magnitude/Round Altitude ==
  note: Round to nearest 100 ft unless desired alt == reference alt and ownship is level
  Alt In : Inport
  Reference Alt : Inport  Port=2
  Ownship Climb/Descend : Inport  Port=3
  Add : Sum
  Compare To Zero : simulink/Logic and Bit Operations/Compare To Zero  relop=~=  OutDataTypeStr=boolean
  Compare To Zero1 : simulink/Logic and Bit Operations/Compare To Zero  relop=~=  OutDataTypeStr=boolean
  Logical Operator : Logic  Operator=OR  AllPortsSameDT=off  OutDataTypeStr=boolean
  Round : Subsystem  mask{factor=100}
      mask prompts: factor "Round to nearest:"
  Scope : Scope
  Scope1 : Scope
  Scope2 : Scope
  Switch1 : Switch  Criteria=u2 > Threshold
  Alt Out : Outport
  wires:
  Compare To Zero1/1 -> Scope/1, Logical Operator/1
  Compare To Zero/1 -> Logical Operator/2, Scope1/1
  Logical Operator/1 -> Switch1/2
  Ownship Climb/Descend/1 -> Compare To Zero1/1
  Switch1/1 -> Alt Out/1
  Reference Alt/1 -> Add/2
  Round/1(Out) -> Switch1/1
  Add/1 -> Round/1(In), Switch1/3, Scope2/1
  Alt In/1 -> Compare To Zero/1, Add/1

== system PilotModelUnitTest/Pilot Model/UAS Pilot Model Release 6.0/Use Pilot Model/Maneuver/Maneuver Selection/Draw Vertical Magnitude/Round Altitude/Round ==
  In : Inport
  Constant : Constant  Value=factor
  Divide : Product  Inputs=*/
  Product : Product
  Rounding Function : Rounding  Operator=round
  Out : Outport
  wires:
  Rounding Function/1 -> Product/1
  In/1 -> Divide/1
  Divide/1 -> Rounding Function/1
  Constant/1 -> Product/2, Divide/2
  Product/1 -> Out/1

== matlab function PilotModelUnitTest/AC - Track Following/Follow Trajectory/Set LLA /MATLAB Function ==
  data: e_ft input; n_ft input; u_ft input; v_ftps input; psi_rad input; theta_rad input; lat0 input; lat_rad output; lon0 input; h0 input; lon_rad output; dlat_radps output; dlon_radps output; alt_ft output; dalt_ftps output
function [lat_rad,lon_rad,dlat_radps,dlon_radps,alt_ft,dalt_ftps] = convertToLLA(e_ft,n_ft,u_ft,v_ftps,psi_rad,theta_rad,lat0,lon0,h0)
%#codegen

% WGS-84 ellipsoid constants
a = 2.09256*10^7;          %Semi-major axis (meters)
f = 1.0/298.257223563;  %Flattening
ecc_sq = f*(2.0-f);        %Eccentricity^2


% Ellipsoidal "radius"
er = a./sqrt(1-ecc_sq.*sin(lat0).^2);


% ECEF coordinates
x0 = (er + h0)*cos(lat0)*cos(lon0);
y0 = (er + h0)*cos(lat0)*sin(lon0);
z0 = (er.*(1-ecc_sq) + h0)*sin(lat0);


%% Rotation Matrix
posECEF0 = [x0;y0;z0];
% Compute the local Up unit vector
vHatU = posECEF0;
vHatU(3) = vHatU(3) ./ ((1-f)^2);
vHatU = vHatU ./ norm(vHatU);

% Compute the projection onto the local Up vector
pU = vHatU * vHatU';

% Compute the projection onto the local Tangent plane
pT = eye(size(pU)) - pU;

% Compute the local North unit vector
vHatZ = [0;0;1];
vHatN = pT * vHatZ;
vHatN = vHatN ./ norm(vHatN);

% Compute the local East unit vector
vHatE = cross(vHatN,vHatU);

% Compute ENU rotation matrix
rotMatENU = zeros(3,3);
rotMatENU(:,1) = vHatE;
rotMatENU(:,2) = vHatN;
rotMatENU(:,3) = vHatU;

tPosECEF = rotMatENU*[e_ft;n_ft;u_ft] + [x0;y0;z0];


%% ECEF to LLA
% WGS-84 derived parameters
b = (1-f).*a;                       %Semi-minor axis (meters)
ecc1_sq = (a.^2 - b.^2)./(a.^2);    %First eccentricity squared
ecc2_sq = (a.^2 - b.^2)./(b.^2);    %Second eccentricity squared


% Length of position vector in equatorial plane
rho = sqrt(tPosECEF(1).^2 + tPosECEF(2).^2);

% Auxillary angle
theta = atan( (tPosECEF(3).*a)./(rho.*b) );

lon_rad = atan2(tPosECEF(2),tPosECEF(1));
lat_rad = atan( (tPosECEF(3) + ecc2_sq.*b.*(sin(theta)).^3)./(rho - ecc1_sq.*a.*(cos(theta)).^3) );

ewRadCurv = a./sqrt(1-ecc1_sq.*sin(lat_rad).^2);

alt_ft = (rho./cos(lat_rad)) - ewRadCurv;


%% Velocities - Project 1 sec into future and use to estimate
dalt_ftps = v_ftps*sin(theta_rad); % Assume about the same


tPosECEF_1sec = rotMatENU*[e_ft+v_ftps*sin(theta_rad)*sin(psi_rad);...
                           n_ft+v_ftps*sin(theta_rad)*cos(psi_rad);...
                           u_ft] + ...
                           [x0;y0;z0];

% Length of position vector in equatorial plane
rho = sqrt(tPosECEF_1sec(1).^2 + tPosECEF_1sec(2).^2);

% Auxillary angle
theta = atan( (tPosECEF_1sec(3).*a)./(rho.*b) );

lon_rad_1sec = atan2(tPosECEF_1sec(2),tPosECEF_1sec(1));
lat_rad_1sec = atan( (tPosECEF_1sec(3) + ecc2_sq.*b.*(sin(theta)).^3)./(rho - ecc1_sq.*a.*(cos(theta)).^3) );

dlat_radps = lat_rad_1sec - lat_rad;
dlon_radps = lon_rad_1sec - lon_rad;
end

== matlab function PilotModelUnitTest/Pilot Model/Horizontal and Vertical guidance enabler/Vertical Band manipulation ==
  data: Guidance_in input; Guidance_out output
function Guidance_out = fcn(Guidance_in)

temp = Guidance_in;
temp(273) = 4;
temp(275) = 4;
temp(277) = 4;
temp(279) = 4;
temp(281) = 4;
%temp(283) = 4;

Guidance_out = temp;

== matlab function PilotModelUnitTest/Pilot Model/Horizontal and Vertical guidance enabler/Horizontal Band manipulation ==
  data: Guidance_in input; Guidance_out output
function Guidance_out = fcn(Guidance_in)

temp = Guidance_in;
temp(1:271) = 4;

Guidance_out = temp;

== matlab function PilotModelUnitTest/Pilot Model/UAS Pilot Model Release 6.0/Use Pilot Model/Maneuver/Coordination Delay/Draw Coord Delay/Generate Random Gamma Deviate/MATLAB Function ==
  data: a input; y output; b input; seed input
function y = fcn(a, b, seed)
%#codegen

info = rng;
if info.Seed ~= seed
  rng(seed);
end

y = HeuristicOperatorModelR6_ExternalFunctions.gammaDeviate(a,b);

== matlab function PilotModelUnitTest/Pilot Model/UAS Pilot Model Release 6.0/Use Pilot Model/Maneuver/Initial Delay/Draw Initial Delay/Generate Random Exponential Deviate/MATLAB Function ==
  data: a input; y output; seed input
function y = fcn(a, seed)
%#codegen

info = rng;
if info.Seed ~= seed
  rng(seed);
end

y = HeuristicOperatorModelR6_ExternalFunctions.exponentialDeviate(a);

== matlab function PilotModelUnitTest/Pilot Model/UAS Pilot Model Release 6.0/Use Pilot Model/Maneuver/Maneuver Selection/Choose Horizontal Maneuver/Minimum Maneuver Heuristic ==
  data: maneuvers input; index output; wc_flags input; preference_min input; preference_dir input; max_diff input; seed input; isMin output
function [index, isMin] = fcn(maneuvers, wc_flags, preference_min, preference_dir, max_diff, seed)
%#codegen

index = 0;
isMin = true;
[index, isMin] = HeuristicOperatorModelR6_ExternalFunctions.chooseMinimumManeuver(maneuvers, wc_flags, preference_min, preference_dir, max_diff, seed);

== matlab function PilotModelUnitTest/Pilot Model/UAS Pilot Model Release 6.0/Use Pilot Model/Maneuver/Maneuver Selection/Choose Maneuver/MATLAB Function ==
  data: preferTurn input; chooseTurn output; turn_flag input; vert_flag input
function chooseTurn = fcn(preferTurn, turn_flag, vert_flag)
%#codegen

chooseTurn = 1; %#ok<NASGU>
chooseTurn = HeuristicOperatorModelR6_ExternalFunctions.chooseBetweenHorzAndVert(preferTurn, turn_flag, vert_flag);

== matlab function PilotModelUnitTest/Pilot Model/UAS Pilot Model Release 6.0/Use Pilot Model/Maneuver/Maneuver Selection/Draw Horizontal Magnitude/MATLAB Function ==
  data: maneuver input; magnitude output; k input; theta input; offset input; seed input
function magnitude = fcn(maneuver, k, theta, offset, seed)
%#codegen

magnitude = HeuristicOperatorModelR6_ExternalFunctions.drawManeuverMagnitude(maneuver, k, theta, offset, seed);

== matlab function PilotModelUnitTest/Pilot Model/UAS Pilot Model Release 6.0/Use Pilot Model/Maneuver/Maneuver Selection/Draw Vertical Magnitude/MATLAB Function ==
  data: maneuver input; magnitude output; k input; theta input; offset input; seed input
function magnitude = fcn(maneuver, k, theta, offset, seed)
%#codegen

magnitude = HeuristicOperatorModelR6_ExternalFunctions.drawManeuverMagnitude(maneuver, k, theta, offset, seed);

== matlab function PilotModelUnitTest/Pilot Model/UAS Pilot Model Release 6.0/Use Pilot Model/Maneuver/Maneuver Selection/Get Minimum Maneuvers/Get Minimum Altitudes ==
  data: bands input; alts output; wc_flag output; currAlt input
function [alts, wc_flag] = fcn(bands, currAlt)
%#codegen

% pre-define output variable
alts = [0; 0]; %#ok<NASGU>
wc_flag = [0; 0]; %#ok<NASGU>

[alts, wc_flag] = HeuristicOperatorModelR6_ExternalFunctions.getMinimumAltitudes(bands, currAlt);

== matlab function PilotModelUnitTest/Pilot Model/UAS Pilot Model Release 6.0/Use Pilot Model/Maneuver/Maneuver Selection/Get Minimum Maneuvers/Get Minimum Turns ==
  data: bands input; turns output; wc_flag output
function [turns, wc_flag] = fcn(bands)
%#codegen

% pre-define output variable
turns = [0; 0]; %#ok<NASGU>
wc_flag = [0; 0]; %#ok<NASGU>

[turns, wc_flag] = HeuristicOperatorModelR6_ExternalFunctions.getMinimumTurns(bands);

== matlab function PilotModelUnitTest/Pilot Model/UAS Pilot Model Release 6.0/Use Pilot Model/Maneuver/Maneuver Selection/Vertical Maneuver Heuristic/Minimum Maneuver Heuristic ==
  data: maneuvers input; index output; wc_flags input; preference_min input; preference_dir input; seed input
function index = fcn(maneuvers, wc_flags, preference_min, preference_dir, seed)
%#codegen

index = 0;
max_diff = 1e6;
index = HeuristicOperatorModelR6_ExternalFunctions.chooseMinimumManeuver(maneuvers, wc_flags, preference_min, preference_dir, max_diff, seed);
